simulink model "arm_copy"  (R2013a)
settings: Solver=FixedStepDiscrete  StartTime=0.0  StopTime=inf  RelTol=1e-3
undefined symbols (not defined in the file): darwinop_communication_setup
libraries: lib_darwinop x1
settings Model: Creator=florent  LastModifiedBy=florent
settings OptimizationCC: OptimizeModelRefInitCode=on  LifeSpan=1
settings HardwareCC: ProdEndianess=LittleEndian  ProdHWDeviceType=Generic->32-bit Embedded Processor
settings RTWCC: SystemTargetFile=darwinoplib.tlc  TemplateMakefile=darwinoplib.tmf  Description=DarwinOP code generator  ProcessScript=darwinoplib_make_rtw_hook  TargetLang=C++
settings CodeAppCC: IgnoreCustomStorageClasses=off
settings STFCustomTargetCC: CombineOutputUpdateFcns=on  ERTCustomFileBanners=on  SupportContinuousTime=off  SupportNonInlinedSFcns=off  MATLABClassNameForMDSCustomization=Simulink.SoftwareTarget.ERTCustomization  SystemTargetFile=darwinoplib.tlc
settings ERTTargetCC: GenerateSampleERTMain=off  ParMdlRefBuildCompliant=off  CompOptLevelCompliant=off  ConcurrentExecutionCompliant=off  ERTFirstTimeCompliant=off  ModelStepFunctionPrototypeControlCompliant=off  CPPClassGenCompliant=off  ERTCustomFileTemplate=darwinoplib_main.tlc

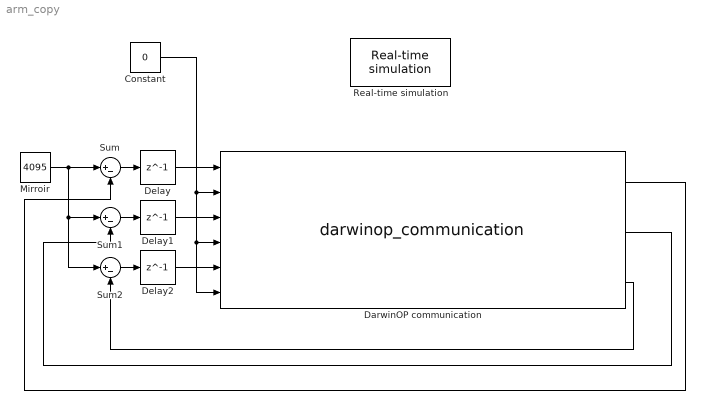
== system arm_copy ==
  Constant : Constant  Value=0
  DarwinOP communication : M-S-Function  StartFcn=darwinop_communication_setup('StartFcn');  StopFcn=darwinop_communication_setup('StopFcn');  FunctionName=darwinop_communication  Parameters=IP,Port,Protocol,Timeout,Frame,ReadIndex,WriteIndex  mask{IP=192.168.123.1, Port=1234, Protocol=tcp, Timeout=0.05, Frame=[ 3 1 30 2 0 0 2 2 36 2 3 2 24 1 0 3 3 30 2 0 0 2 4 36 2 3 4 24 1 0 3 5 30 2 0 0 2 6 36 2 3 6 24 1 0], ReadIndex=[ 1 2;3 2;5 2], WriteIndex=[ 5 2;15 1;20 2;30 1;35 2;45 1]}
      settings: DeleteFcn=darwinop_communication_setup('DeleteFcn');  ModelCloseFcn=darwinop_communication_setup('ModelCloseFcn');  NameChangeFcn=darwinop_communication_setup('NameChangeFcn');  OpenFcn=darwinop_communication_setup('OpenFcn');
      mask TypeOptions Protocol: tcp | udp
      mask Display:
      | image('darwin-blk.jpg')
      | 
      | port_label('output',1,'Left Shoulder Pitch(2)/Position')
      | port_label('output',2,'Left Shoulder Roll(4)/Position')
      | port_label('output',3,'Left Elbow(6)/Position')
      | 
      | port_label('input',1,'Right Shoulder Pitch(1)/Goal Position')
      | port_label('input',2,'Left Shoulder Pitch(2)/Torque Enable')
      | port_label('input',3,'Right Shoulder Roll(3)/Goal Position')
      | port_label('input',4,'Left Shoulder Roll(4)/Torque Enable')
      | port_label('input',5,'Right Elbow(5)/Goal Position')
      | port_label('input',6,'Left Elbow(6)/Torque Enable')
  Delay : Delay  DelayLength=1  InitialCondition=2048
  Delay1 : Delay  DelayLength=1  InitialCondition=2048
  Delay2 : Delay  DelayLength=1  InitialCondition=2048
  Mirroir : Constant  Value=4095
  Real-time simulation : lib_darwinop/Real-time simulation  TimeScalingFactor=1
  Sum : Sum  Inputs=|+-
  Sum1 : Sum  Inputs=|+-
  Sum2 : Sum  Inputs=|+-
  wires:
  Sum2/1 -> Delay2/1
  Sum1/1 -> Delay1/1
  Sum/1 -> Delay/1
  Mirroir/1 -> Sum2/1, Sum1/1, Sum/1
  DarwinOP communication/1 -> Sum/2
  DarwinOP communication/2 -> Sum1/2
  DarwinOP communication/3 -> Sum2/2
  Constant/1 -> DarwinOP communication/6, DarwinOP communication/4, DarwinOP communication/2
  Delay/1 -> DarwinOP communication/1
  Delay1/1 -> DarwinOP communication/3
  Delay2/1 -> DarwinOP communication/5
